simulink model "Example_InterfaceToUSV"  (R2024a)
settings: Solver=FixedStepAuto  StartTime=0.0  StopTime=inf  FixedStep=0.01  RelTol=1e-3
undefined symbols (not defined in the file): actuatorCommand, allocationCommand, commandMode, ready, timestampUTC, useXNAllocation
libraries: MESSIN_Library x3, simulink_extras x2
settings Model: Creator=Scythe  LastModifiedBy=Scythe
settings SolverCC: ConcurrentTasks=on
settings DataIOCC: SaveOutput=off  SignalLogging=off  DSMLogging=off  SaveTime=off  ReturnWorkspaceOutputs=off
settings OptimizationCC: DefaultParameterBehavior=Inlined  ZeroExternalMemoryAtStartup=off  ZeroInternalMemoryAtStartup=off  SimCompilerOptimization=on
settings DebuggingCC: UnconnectedInputMsg=warning  UnconnectedOutputMsg=warning  UnconnectedLineMsg=warning
settings HardwareCC: ProdBitPerLong=64  ProdHWDeviceType=Intel->x86-64 (Linux 64)
settings ModelReferenceCC: EnableRefExpFcnMdlSchedulingChecks=on
settings SFSimCC: SimParseCustomCode=off  SimGenImportedTypeDefs=on  SimTargetLang=C++
settings RTWCC: GenCodeOnly=on  PackageGeneratedCodeAndArtifacts=on  PackageName=PackNGo  RTWVerbose=off  BuildConfiguration=Faster Runs  TargetLang=C++
settings CodeAppCC: ForceParamTrailComments=on  MaxIdLength=128  StateflowObjectComments=on  MATLABSourceComments=on  UseSimReservedNames=on
settings GRTTargetCC: TargetLangStandard=C++11 (ISO)  MatFileLogging=off  CodeInterfacePackaging=C++ class

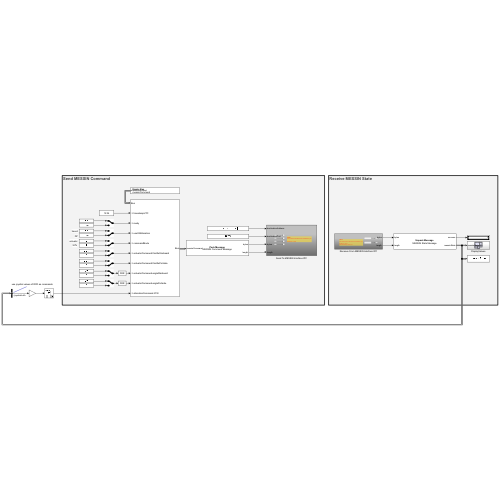
[thumbnail: Simulink's stored preview of the top-level diagram]
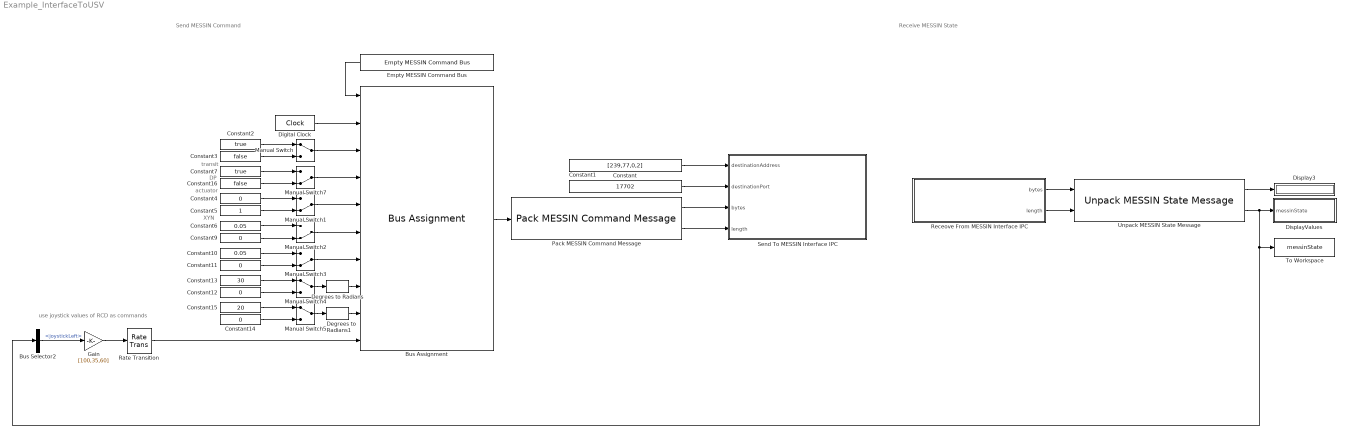
== system Example_InterfaceToUSV ==
  note: use joystick values of RCD as commands
  note: actuator
  note: Receive MESSIN State
  note: XYN
  note: Send MESSIN Command
  note: transit
  note: DP
  Bus Assignment : BusAssignment  AssignedSignals=timestampUTC,ready,useXNAllocation,commandMode,actuatorCommand.throttleStarboard,actuatorCommand.throttlePortside,actuatorCommand.angleStarboard,actuatorCommand.anglePortside,allocationCommand.XYN
  Bus Selector2 : BusSelector  OutputSignals=remoteControlDevice.joystickLeft
  Constant : Constant  Value=[239,77,0,2]  OutDataTypeStr=uint8
  Constant1 : Constant  Value=17702  OutDataTypeStr=uint16
  Constant10 : Constant  Value=0.05  OutDataTypeStr=double
  Constant{9,11..12,14} (4 alike) : Constant  Value=0  OutDataTypeStr=double
  Constant13 : Constant  Value=30  OutDataTypeStr=double
  Constant15 : Constant  Value=20  OutDataTypeStr=double
  Constant16 : Constant  Value=false  OutDataTypeStr=boolean
  Constant2 : Constant  Value=true  OutDataTypeStr=boolean
  Constant3 : Constant  Value=false  OutDataTypeStr=boolean
  Constant4 : Constant  Value=0  OutDataTypeStr=uint8
  Constant5 : Constant  OutDataTypeStr=uint8
  Constant6 : Constant  Value=0.05  OutDataTypeStr=double
  Constant7 : Constant  Value=true  OutDataTypeStr=boolean
  Degrees to Radians : simulink_extras/Transformations/Degrees to Radians
  Degrees to Radians1 : simulink_extras/Transformations/Degrees to Radians
  Digital Clock : DigitalClock  SampleTime=0.1
  Display3 : Display
  DisplayValues : Subsystem
  Empty MESSIN Command Bus : MESSIN_Library/Command Message/Empty MESSIN Command Bus
      settings: SourceProductName=MESSIN - Interface Library
  Gain : Gain  Gain=[100,35,60]
  Manual Switch : ManualSwitch
  Manual Switch{1..3,7} (4 alike) : ManualSwitch  CurrentSetting=0
  Manual Switch4 : ManualSwitch
  Manual Switch5 : ManualSwitch
  Pack MESSIN Command Message : MESSIN_Library/Command Message/Pack MESSIN Command Message
      settings: SourceProductName=MESSIN - Interface Library
  Rate Transition : RateTransition  Deterministic=off  OutPortSampleTime=0.1
  Receove From MESSIN Interface IPC : Subsystem
  Send To MESSIN Interface IPC : Subsystem
  To Workspace : ToWorkspace  VariableName=messinState  SaveFormat=Timeseries  SampleTime=-1
  Unpack MESSIN State Message : MESSIN_Library/State Message/Unpack MESSIN State Message
      settings: SourceProductName=MESSIN - Interface Library
  wires:
  Manual Switch7/1 -> Bus Assignment/4
  Constant7/1 -> Manual Switch7/1
  Constant16/1 -> Manual Switch7/2
  Rate Transition/1 -> Bus Assignment/10
  Bus Selector2/1 -> Gain/1  "<joystickLeft>"
  Unpack MESSIN State Message/2 -> DisplayValues/1(messinState), Bus Selector2/1, To Workspace/1
  Gain/1 -> Rate Transition/1
  Manual Switch5/1 -> Degrees to Radians1/1
  Constant14/1 -> Manual Switch5/2
  Constant15/1 -> Manual Switch5/1
  Degrees to Radians1/1 -> Bus Assignment/9
  Degrees to Radians/1 -> Bus Assignment/8
  Constant13/1 -> Manual Switch4/1
  Constant12/1 -> Manual Switch4/2
  Manual Switch4/1 -> Degrees to Radians/1
  Manual Switch3/1 -> Bus Assignment/7
  Constant10/1 -> Manual Switch3/1
  Constant11/1 -> Manual Switch3/2
  Constant9/1 -> Manual Switch2/2
  Constant6/1 -> Manual Switch2/1
  Manual Switch2/1 -> Bus Assignment/6
  Constant5/1 -> Manual Switch1/2
  Constant4/1 -> Manual Switch1/1
  Manual Switch1/1 -> Bus Assignment/5
  Constant3/1 -> Manual Switch/2
  Constant2/1 -> Manual Switch/1
  Manual Switch/1 -> Bus Assignment/3
  Digital Clock/1 -> Bus Assignment/2
  Bus Assignment/1 -> Pack MESSIN Command Message/1
  Empty MESSIN Command Bus/1 -> Bus Assignment/1
  Pack MESSIN Command Message/1 -> Send To MESSIN Interface IPC/3(bytes)
  Constant1/1 -> Send To MESSIN Interface IPC/2(destinationPort)
  Constant/1 -> Send To MESSIN Interface IPC/1(destinationAddress)
  Unpack MESSIN State Message/1 -> Display3/1
  Receove From MESSIN Interface IPC/2(length) -> Unpack MESSIN State Message/2
  Receove From MESSIN Interface IPC/1(bytes) -> Unpack MESSIN State Message/1
  Pack MESSIN Command Message/2 -> Send To MESSIN Interface IPC/4(length)

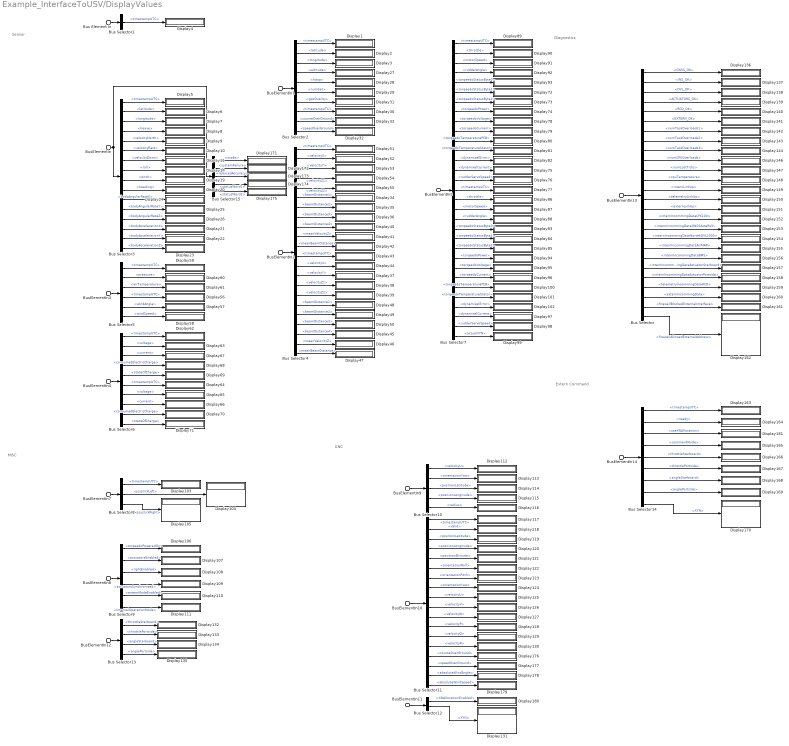
== system Example_InterfaceToUSV/DisplayValues ==
  note: Sensor
  note: GNC
  note: MISC
  note: Extern Command
  note: Diagnostics
  Bus Element In : Inport  PortName=messinState
  BusElementIn : Inport  PortName=messinState  Element=sensor.insLFK100
  BusElementIn1 : Inport  PortName=messinState  Element=sensor.gnssAsteRx3
  BusElementIn2 : Inport  PortName=messinState  Element=sensor.nortekDVL1000
  BusElementIn3 : Inport  PortName=messinState  Element=sensor.airMAR
  BusElementIn4 : Inport  PortName=messinState  Element=sensor.batteryManagementSystem
  BusElementIn5 : Inport  PortName=messinState  Element=sensor.messinDrive
  BusElementIn7 : Inport  PortName=messinState  Element=remoteControlDevice
  BusElementIn8 : Inport  PortName=messinState  Element=supervisor
  BusElementIn9 : Inport  PortName=messinState  Element=gnc.guidance
  BusElementIn10 : Inport  PortName=messinState  Element=gnc.navigation
  BusElementIn11 : Inport  PortName=messinState  Element=gnc.control
  BusElementIn12 : Inport  PortName=messinState  Element=commandedActuator
  BusElementIn13 : Inport  PortName=messinState  Element=systemDiagnostics
  BusElementIn14 : Inport  PortName=messinState  Element=externCommand
  Bus Selector : BusSelector  OutputSignals=GNSS_OK,INS_OK,DVL_OK,ACTUATORS_OK,RCD_OK,EXTERN_OK,details.hardware.numTaskOverloads1,details.hardware.numTaskOverloads2,details.hardware.numTaskOverloads3,details.hardware.numCPUOverloads,details.hardware.numLostTicks,details.hardware.cpuTemperature,details.network.internLinkUp,details.network.telemetryLinkUp,details.network.externLinkUp,details.network.internIncommingDataLFK100,details.network.internIncommingDataGNSSAsteRx3,details.network.internIncommingDataNortekDVL1000,details.network.internIncommingDataAirMAR,details.network.internIncommingDataBMS,details.network.internIncommingDataActuatorStarboard,details.network.internIncommingDataActuatorPortside,details.network.telemetryIncommingDataRCD,details.network.externIncommingData,details.network.firewallBlockedExternalInterface,details.network.firewallAllowedExternalAddress
  Bus Selector1 : BusSelector  OutputSignals=timestampUTC
  Bus Selector10 : BusSelector  OutputSignals=surgeHeading.velocityU,surgeHeading.orientationYaw,stayThere.positionLatitude,stayThere.positionLongitude,stayThere.radius
  Bus Selector11 : BusSelector  OutputSignals=timestampUTC,info.valid,state.positionLatitude,state.positionLongitude,state.positionAltitude,state.orientationRoll,state.orientationPitch,state.orientationYaw,state.velocityU,state.velocityV,state.velocityW,state.velocityP,state.velocityQ,state.velocityR,state.courseOverGround,state.speedOverGround,state.absoluteWindAngle,state.absoluteWindSpeed
  Bus Selector12 : BusSelector  OutputSignals=XNAllocationEnabled,XYN
  Bus Selector13 : BusSelector  OutputSignals=throttleStarboard,throttlePortside,angleStarboard,anglePortside
  Bus Selector14 : BusSelector  OutputSignals=timestampUTC,ready,useXNAllocation,commandMode,actuatorCommand.throttleStarboard,actuatorCommand.throttlePortside,actuatorCommand.angleStarboard,actuatorCommand.anglePortside,allocationCommand.XYN
  Bus Selector15 : BusSelector  OutputSignals=details.mode,details.systemFailure,details.reducedAccuracy,details.statusWord1,details.statusWord2
  Bus Selector2 : BusSelector  OutputSignals=gnss.timestampUTC,gnss.latitude,gnss.longitude,gnss.altitude,gnss.hdop,gnss.numSat,gnss.gpsQuality,courseAndSpeedOverGround.timestampUTC,courseAndSpeedOverGround.courseOverGround,courseAndSpeedOverGround.speedOverGround
  Bus Selector3 : BusSelector  OutputSignals=timestampUTC,latitude,longitude,heave,velocityNorth,velocityEast,velocityDown,roll,pitch,heading,bodyAngularRateX,bodyAngularRateY,bodyAngularRateZ,bodyAccelerationX,bodyAccelerationY,bodyAccelerationZ
  Bus Selector4 : BusSelector  OutputSignals=bottomTrack.timestampUTC,bottomTrack.velocityX,bottomTrack.velocityY,bottomTrack.velocityZ1,bottomTrack.velocityZ2,bottomTrack.beamDistance1,bottomTrack.beamDistance2,bottomTrack.beamDistance3,bottomTrack.beamDistance4,bottomTrack.meanVelocityZ,bottomTrack.meanBeamDistance,waterTrack.timestampUTC,waterTrack.velocityX,waterTrack.velocityY,waterTrack.velocityZ1,waterTrack.velocityZ2,waterTrack.beamDistance1,waterTrack.beamDistance2,waterTrack.beamDistance3,waterTrack.beamDistance4,waterTrack.meanVelocityZ,waterTrack.meanBeamDistance
  Bus Selector5 : BusSelector  OutputSignals=air.timestampUTC,air.pressure,air.airTemperature,relativeWind.timestampUTC,relativeWind.windAngle,relativeWind.windSpeed
  Bus Selector6 : BusSelector  OutputSignals=batteryStarboard.timestampUTC,batteryStarboard.voltage,batteryStarboard.current,batteryStarboard.consumedElectricCharge,batteryStarboard.stateOfCharge,batteryPortside.timestampUTC,batteryPortside.voltage,batteryPortside.current,batteryPortside.consumedElectricCharge,batteryPortside.stateOfCharge
  Bus Selector7 : BusSelector  OutputSignals=actuatorStarboard.timestampUTC,actuatorStarboard.throttle,actuatorStarboard.motorSpeed,actuatorStarboard.rudderAngle,actuatorStarboard.torqeedoStatusByte0,actuatorStarboard.torqeedoStatusByte1,actuatorStarboard.torqeedoStatusByte2,actuatorStarboard.torqeedoPower,actuatorStarboard.torqeedoVoltage,actuatorStarboard.torqeedoCurrent,actuatorStarboard.torqeedoTemperaturePCB,actuatorStarboard.torqeedoTemperatureStator,actuatorStarboard.dynamixelError,actuatorStarboard.dynamixelCurrent,actuatorStarboard.rudderServoSpeed,actuatorPortside.timestampUTC,actuatorPortside.throttle,actuatorPortside.motorSpeed,actuatorPortside.rudderAngle,actuatorPortside.torqeedoStatusByte0,actuatorPortside.torqeedoStatusByte1,actuatorPortside.torqeedoStatusByte2,actuatorPortside.torqeedoPower,actuatorPortside.torqeedoVoltage,actuatorPortside.torqeedoCurrent,actuatorPortside.torqeedoTemperaturePCB,actuatorPortside.torqeedoTemperatureStator,actuatorPortside.dynamixelError,actuatorPortside.dynamixelCurrent,actuatorPortside.rudderServoSpeed,actualXYN
  Bus Selector8 : BusSelector  OutputSignals=timestampUTC,joystickLeft,joystickRight
  Bus Selector9 : BusSelector  OutputSignals=torqeedoPoweredOn,actuatorsEnabled,lightEnabled,actuatorsSynchronized,externModeEnabled,internalOperationMode
  Display{1..11,18..144,146..181} (174 alike) : Display
  wires:
  Bus Selector14/3 -> Display181/1  "<useXNAllocation>"
  Bus Selector12/1 -> Display180/1  "<XNAllocationEnabled>"
  Bus Selector11/15 -> Display176/1  "<courseOverGround>"
  Bus Selector11/16 -> Display177/1  "<speedOverGround>"
  Bus Selector11/18 -> Display179/1  "<absoluteWindSpeed>"
  Bus Selector11/17 -> Display178/1  "<absoluteWindAngle>"
  Bus Selector15/5 -> Display175/1  "<statusWord2>"
  Bus Selector15/4 -> Display174/1  "<statusWord1>"
  Bus Selector15/3 -> Display173/1  "<reducedAccuracy>"
  Bus Selector15/2 -> Display172/1  "<systemFailure>"
  Bus Selector15/1 -> Display171/1  "<mode>"
  Bus Selector14/6 -> Display167/1  "<throttlePortside>"
  Bus Selector14/7 -> Display168/1  "<angleStarboard>"
  Bus Selector14/9 -> Display170/1  "<XYN>"
  Bus Selector14/8 -> Display169/1  "<anglePortside>"
  Bus Selector14/4 -> Display165/1  "<commandMode>"
  Bus Selector14/5 -> Display166/1  "<throttleStarboard>"
  Bus Selector14/2 -> Display164/1  "<ready>"
  Bus Selector14/1 -> Display163/1  "<timestampUTC>"
  BusElementIn14/1 -> Bus Selector14/1
  Bus Selector/16 -> Display152/1  "<internIncommingDataLFK100>"
  Bus Selector/17 -> Display153/1  "<internIncommingDataGNSSAsteRx3>"
  Bus Selector/19 -> Display155/1  "<internIncommingDataAirMAR>"
  Bus Selector/18 -> Display154/1  "<internIncommingDataNortekDVL1000>"
  Bus Selector/22 -> Display158/1  "<internIncommingDataActuatorPortside>"
  Bus Selector/23 -> Display159/1  "<telemetryIncommingDataRCD>"
  Bus Selector/21 -> Display157/1  "<internIncommingDataActuatorStarboard>"
  Bus Selector/20 -> Display156/1  "<internIncommingDataBMS>"
  Bus Selector/26 -> Display162/1  "<firewallAllowedExternalAddress>"
  Bus Selector/25 -> Display161/1  "<firewallBlockedExternalInterface>"
  Bus Selector/24 -> Display160/1  "<externIncommingData>"
  Bus Selector/9 -> Display144/1  "<numTaskOverloads3>"
  Bus Selector/11 -> Display147/1  "<numLostTicks>"
  Bus Selector/10 -> Display146/1  "<numCPUOverloads>"
  Bus Selector/14 -> Display150/1  "<telemetryLinkUp>"
  Bus Selector/15 -> Display151/1  "<externLinkUp>"
  Bus Selector/13 -> Display149/1  "<internLinkUp>"
  Bus Selector/12 -> Display148/1  "<cpuTemperature>"
  Bus Selector/5 -> Display140/1  "<RCD_OK>"
  Bus Selector/6 -> Display141/1  "<EXTERN_OK>"
  Bus Selector/8 -> Display143/1  "<numTaskOverloads2>"
  Bus Selector/7 -> Display142/1  "<numTaskOverloads1>"
  Bus Selector/3 -> Display138/1  "<DVL_OK>"
  Bus Selector/4 -> Display139/1  "<ACTUATORS_OK>"
  Bus Selector/2 -> Display137/1  "<INS_OK>"
  Bus Selector/1 -> Display136/1  "<GNSS_OK>"
  BusElementIn13/1 -> Bus Selector/1
  Bus Selector13/3 -> Display134/1  "<angleStarboard>"
  Bus Selector13/4 -> Display135/1  "<anglePortside>"
  Bus Selector13/2 -> Display133/1  "<throttlePortside>"
  Bus Selector13/1 -> Display132/1  "<throttleStarboard>"
  BusElementIn12/1 -> Bus Selector13/1
  Bus Selector12/2 -> Display131/1  "<XYN>"
  BusElementIn11/1 -> Bus Selector12/1
  Bus Selector11/13 -> Display129/1  "<velocityQ>"
  Bus Selector11/14 -> Display130/1  "<velocityR>"
  Bus Selector11/7 -> Display123/1  "<orientationPitch>"
  Bus Selector11/12 -> Display128/1  "<velocityP>"
  Bus Selector11/10 -> Display126/1  "<velocityV>"
  Bus Selector11/11 -> Display127/1  "<velocityW>"
  Bus Selector11/9 -> Display125/1  "<velocityU>"
  Bus Selector11/8 -> Display124/1  "<orientationYaw>"
  Bus Selector11/2 -> Display118/1  "<valid>"
  Bus Selector11/3 -> Display119/1  "<positionLatitude>"
  Bus Selector11/5 -> Display121/1  "<positionAltitude>"
  Bus Selector11/4 -> Display120/1  "<positionLongitude>"
  Bus Selector11/6 -> Display122/1  "<orientationRoll>"
  Bus Selector11/1 -> Display117/1  "<timestampUTC>"
  BusElementIn10/1 -> Bus Selector11/1
  Bus Selector10/5 -> Display116/1  "<radius>"
  Bus Selector10/3 -> Display114/1  "<positionLatitude>"
  Bus Selector10/4 -> Display115/1  "<positionLongitude>"
  Bus Selector10/2 -> Display113/1  "<orientationYaw>"
  Bus Selector10/1 -> Display112/1  "<velocityU>"
  BusElementIn9/1 -> Bus Selector10/1
  Bus Selector9/6 -> Display111/1  "<internalOperationMode>"
  Bus Selector9/5 -> Display110/1  "<externModeEnabled>"
  Bus Selector9/3 -> Display108/1  "<lightEnabled>"
  Bus Selector9/4 -> Display109/1  "<actuatorsSynchronized>"
  Bus Selector9/2 -> Display107/1  "<actuatorsEnabled>"
  Bus Selector9/1 -> Display106/1  "<torqeedoPoweredOn>"
  BusElementIn8/1 -> Bus Selector9/1
  Bus Selector8/3 -> Display105/1  "<joystickRight>"
  Bus Selector8/2 -> Display104/1  "<joystickLeft>"
  Bus Selector8/1 -> Display103/1  "<timestampUTC>"
  BusElementIn7/1 -> Bus Selector8/1
  Bus Selector7/30 -> Display98/1  "<rudderServoSpeed>"
  Bus Selector7/28 -> Display102/1  "<dynamixelError>"
  Bus Selector7/27 -> Display101/1  "<torqeedoTemperatureStator>"
  Bus Selector7/25 -> Display96/1  "<torqeedoCurrent>"
  Bus Selector7/26 -> Display100/1  "<torqeedoTemperaturePCB>"
  Bus Selector7/23 -> Display94/1  "<torqeedoPower>"
  Bus Selector7/29 -> Display97/1  "<dynamixelCurrent>"
  Bus Selector7/24 -> Display95/1  "<torqeedoVoltage>"
  Bus Selector7/31 -> Display99/1  "<actualXYN>"
  Bus Selector7/12 -> Display81/1  "<torqeedoTemperatureStator>"
  Bus Selector7/22 -> Display85/1  "<torqeedoStatusByte2>"
  Bus Selector7/1 -> Display89/1  "<timestampUTC>"
  Bus Selector7/11 -> Display80/1  "<torqeedoTemperaturePCB>"
  Bus Selector7/6 -> Display72/1  "<torqeedoStatusByte1>"
  Bus Selector7/9 -> Display78/1  "<torqeedoVoltage>"
  Bus Selector7/3 -> Display91/1  "<motorSpeed>"
  Bus Selector7/10 -> Display79/1  "<torqeedoCurrent>"
  Bus Selector7/7 -> Display73/1  "<torqeedoStatusByte2>"
  Bus Selector7/8 -> Display74/1  "<torqeedoPower>"
  Bus Selector7/15 -> Display76/1  "<rudderServoSpeed>"
  Bus Selector7/2 -> Display90/1  "<throttle>"
  Bus Selector7/20 -> Display83/1  "<torqeedoStatusByte0>"
  Bus Selector7/13 -> Display82/1  "<dynamixelError>"
  Bus Selector7/14 -> Display75/1  "<dynamixelCurrent>"
  Bus Selector7/17 -> Display86/1  "<throttle>"
  Bus Selector7/16 -> Display77/1  "<timestampUTC>"
  Bus Selector7/18 -> Display87/1  "<motorSpeed>"
  Bus Selector7/5 -> Display93/1  "<torqeedoStatusByte0>"
  Bus Selector7/4 -> Display92/1  "<rudderAngle>"
  Bus Selector7/19 -> Display88/1  "<rudderAngle>"
  Bus Selector7/21 -> Display84/1  "<torqeedoStatusByte1>"
  BusElementIn5/1 -> Bus Selector7/1
  Bus Selector6/10 -> Display71/1  "<stateOfCharge>"
  Bus Selector6/9 -> Display70/1  "<consumedElectricCharge>"
  Bus Selector6/7 -> Display65/1  "<voltage>"
  Bus Selector6/5 -> Display69/1  "<stateOfCharge>"
  Bus Selector6/4 -> Display68/1  "<consumedElectricCharge>"
  Bus Selector6/2 -> Display63/1  "<voltage>"
  Bus Selector6/3 -> Display67/1  "<current>"
  Bus Selector6/6 -> Display64/1  "<timestampUTC>"
  Bus Selector6/1 -> Display62/1  "<timestampUTC>"
  Bus Selector6/8 -> Display66/1  "<current>"
  BusElementIn4/1 -> Bus Selector6/1
  Bus Selector5/5 -> Display57/1  "<windAngle>"
  Bus Selector5/3 -> Display61/1  "<airTemperature>"
  Bus Selector5/2 -> Display60/1  "<pressure>"
  Bus Selector5/1 -> Display59/1  "<timestampUTC>"
  Bus Selector5/4 -> Display56/1  "<timestampUTC>"
  Bus Selector5/6 -> Display58/1  "<windSpeed>"
  BusElementIn3/1 -> Bus Selector5/1
  Bus Selector4/21 -> Display46/1  "<meanVelocityZ>"
  Bus Selector4/19 -> Display50/1  "<beamDistance3>"
  Bus Selector4/4 -> Display54/1  "<velocityZ1>"
  Bus Selector4/5 -> Display55/1  "<velocityZ2>"
  Bus Selector4/18 -> Display49/1  "<beamDistance2>"
  Bus Selector4/16 -> Display39/1  "<velocityZ2>"
  Bus Selector4/17 -> Display48/1  "<beamDistance1>"
  Bus Selector4/14 -> Display37/1  "<velocityY>"
  Bus Selector4/13 -> Display44/1  "<velocityX>"
  Bus Selector4/20 -> Display45/1  "<beamDistance4>"
  Bus Selector4/2 -> Display52/1  "<velocityX>"
  Bus Selector4/15 -> Display38/1  "<velocityZ1>"
  Bus Selector4/8 -> Display36/1  "<beamDistance3>"
  Bus Selector4/7 -> Display35/1  "<beamDistance2>"
  Bus Selector4/10 -> Display41/1  "<meanVelocityZ>"
  Bus Selector4/3 -> Display53/1  "<velocityY>"
  Bus Selector4/9 -> Display40/1  "<beamDistance4>"
  Bus Selector4/6 -> Display34/1  "<beamDistance1>"
  Bus Selector4/11 -> Display42/1  "<meanBeamDistance>"
  Bus Selector4/1 -> Display51/1  "<timestampUTC>"
  Bus Selector4/22 -> Display47/1  "<meanBeamDistance>"
  Bus Selector4/12 -> Display43/1  "<timestampUTC>"
  BusElementIn2/1 -> Bus Selector4/1
  Bus Selector2/9 -> Display33/1  "<courseOverGround>"
  Bus Selector2/10 -> Display32/1  "<speedOverGround>"
  Bus Selector2/5 -> Display28/1  "<hdop>"
  Bus Selector2/6 -> Display29/1  "<numSat>"
  Bus Selector2/8 -> Display30/1  "<timestampUTC>"
  Bus Selector2/7 -> Display31/1  "<gpsQuality>"
  Bus Selector2/3 -> Display3/1  "<longitude>"
  Bus Selector2/4 -> Display27/1  "<altitude>"
  Bus Selector2/2 -> Display2/1  "<latitude>"
  Bus Selector2/1 -> Display1/1  "<timestampUTC>"
  BusElementIn1/1 -> Bus Selector2/1
  BusElementIn/1 -> Bus Selector3/1, Bus Selector15/1
  Bus Element In/1 -> Bus Selector1/1
  Bus Selector3/9 -> Display19/1  "<pitch>"
  Bus Selector3/16 -> Display23/1  "<bodyAccelerationZ>"
  Bus Selector3/1 -> Display5/1  "<timestampUTC>"
  Bus Selector3/8 -> Display18/1  "<roll>"
  Bus Selector3/6 -> Display10/1  "<velocityEast>"
  Bus Selector3/3 -> Display7/1  "<longitude>"
  Bus Selector1/1 -> Display4/1  "<timestampUTC>"
  Bus Selector3/7 -> Display11/1  "<velocityDown>"
  Bus Selector3/2 -> Display6/1  "<latitude>"
  Bus Selector3/14 -> Display21/1  "<bodyAccelerationX>"
  Bus Selector3/10 -> Display20/1  "<heading>"
  Bus Selector3/11 -> Display24/1  "<bodyAngularRateX>"
  Bus Selector3/12 -> Display25/1  "<bodyAngularRateY>"
  Bus Selector3/5 -> Display9/1  "<velocityNorth>"
  Bus Selector3/4 -> Display8/1  "<heave>"
  Bus Selector3/13 -> Display26/1  "<bodyAngularRateZ>"
  Bus Selector3/15 -> Display22/1  "<bodyAccelerationY>"

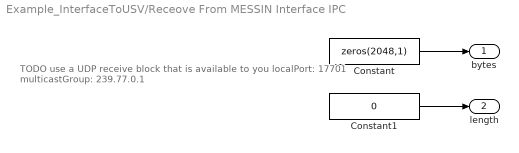
== system Example_InterfaceToUSV/Receove From MESSIN Interface IPC ==
  note: TODO
      | use a UDP receive block that is available to you
      |
      | localPort: 17701
      | multicastGroup: 239.77.0.1
  Constant : Constant  Value=zeros(2048,1)  OutDataTypeStr=uint8
  Constant1 : Constant  Value=0  OutDataTypeStr=uint32
  bytes : Outport
  length : Outport  Port=2
  wires:
  Constant/1 -> bytes/1
  Constant1/1 -> length/1

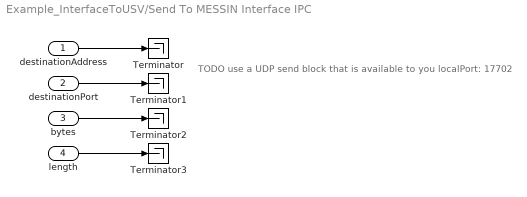
== system Example_InterfaceToUSV/Send To MESSIN Interface IPC ==
  note: TODO
      | use a UDP send block that is available to you
      |
      | localPort: 17702
  destinationAddress : Inport
  destinationPort : Inport  Port=2
  bytes : Inport  Port=3
  length : Inport  Port=4
  Terminator{,1..3} (4 alike) : Terminator
  wires:
  destinationAddress/1 -> Terminator/1
  destinationPort/1 -> Terminator1/1
  bytes/1 -> Terminator2/1
  length/1 -> Terminator3/1
